simulink model "pmuReplay"  (R2018b)
settings: Solver=ode23tb  StartTime=0.0  StopTime=50  MaxStep=1/60  RelTol=1e-4  AbsTol=1e-3  EnableMultiTasking=on
PreLoadFcn:
  | addpath('PMU_Events');
  | load('PMU_ImportedData.mat')
InitFcn:
  | i = 3;
undefined symbols (not defined in the file): D1, Delta
libraries: powerlib x4, simulink x4, microgridLibrary x1, re_lib x1, powerlib_meascontrol x1
Description:
  | Copyright 2008-2017 The MathWorks, Inc.
settings Model: ExtModeAutoUpdateStatusClock=off  Creator=MathWorks  LastModifiedBy=jlesage
settings SolverCC: AutoScaleAbsTol=off
settings DataIOCC: LimitDataPoints=on  SaveFormat=StructureWithTime  SignalLoggingSaveFormat=ModelDataLogs  SaveOutput=off  SignalLogging=off  DSMLogging=off  SaveTime=off  SignalLoggingName=sigsOut
settings OptimizationCC: ExpressionDepthLimit=2147483647  InitFltsAndDblsToZero=on  EfficientMapNaN2IntZero=off  LifeSpan=inf
settings DebuggingCC: UnderspecifiedInitializationDetection=Classic  MergeDetectMultiDrivingBlocksExec=none  CheckExecutionContextPreStartOutputMsg=on  CheckExecutionContextRuntimeOutputMsg=on  SignalResolutionControl=TryResolveAllWithWarning  MultiTaskDSMMsg=warning  MultiTaskCondExecSysMsg=none  FcnCallInpInsideContextMsg=warning  UnconnectedLineMsg=none  StateNameClashWarn=warning  InitInArrayFormatMsg=none  SFUnexpectedBacktrackingDiag=warning  SFNoUnconditionalDefaultTransitionDiag=warning  SFExecutionAtInitializationDiag=none
settings HardwareCC: ProdBitPerPointer=32  ProdBitPerSizeT=32  ProdBitPerPtrDiffT=32  ProdLargestAtomicFloat=None  ProdIntDivRoundTo=Undefined  ProdEndianess=Unspecified  ProdWordSize=32  ProdHWDeviceType=32-bit Generic  TargetUnknown=on
settings ModelReferenceCC: PropagateSignalLabelsOutOfModel=off
settings SFSimCC: SimUseLocalCustomCode=off
settings RTWCC: RTWUseLocalCustomCode=off
settings CodeAppCC: StateflowObjectComments=on
settings GRTTargetCC: TargetLangStandard=C89/C90 (ANSI)  GeneratePreprocessorConditionals=Disable all  CombineOutputUpdateFcns=off  GRTInterface=on
settings ConfigComp: CovMetricSettings=dw  CovHtmlReporting=on  CovSaveCumulativeToWorkspaceVar=on  CovSaveSingleToWorkspaceVar=on  CovExternalEMLEnable=off  CovSFcnEnable=off
settings SimscapeCC: SimscapeNormalizeSystem=off

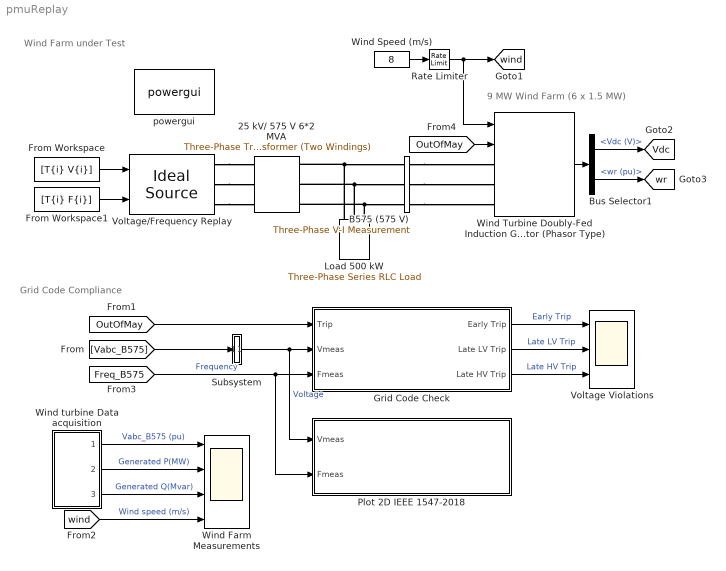
== system pmuReplay ==
  note: Wind Farm under Test
  note: Grid Code Compliance
  note: 9 MW Wind Farm
      | (6 x 1.5 MW)
  25 kV/ 575 V 6*2 MVA : powerlib/Elements/Three-Phase Transformer (Two Windings)  Winding1Connection=Yg  Winding2Connection=Delta (D1)  CoreType=Three single-phase transformers  SetSaturation=off  Hysteresis=off  DataFile='hysteresis'  SetInitialFlux=off  Measurements=None  UNITS=pu  NominalPower="[2e6*6  60]"  Winding1=[25e3 , 0.025/30 , 0.025]  Winding2=[ 575, 0.025/30 , 0.025]  Rm=500  Lm=inf  L0=0.5  Saturation=[ 0,0 ; 0.0024,1.2 ; 1.0,1.52 ]  InitialFluxes=[ 0.8 , -0.8 , 0.7 ]  MoreParameters=off  BreakLoop=off  DataType=off  TransfoNumber=0
      settings: SourceProductName=Simscape Electrical
  B575 (575 V) : powerlib/Measurements/Three-Phase V-I Measurement  VoltageMeasurement=phase-to-ground  SetLabelV=on  LabelV=Vabc_B575  Vpu=on  VpuLL=off  CurrentMeasurement=yes  SetLabelI=on  LabelI=Iabc_B575  Ipu=on  Pbase=6*1.5e6/0.9  Vbase=575  OutputType=Complex  PhasorSimulation=on  PSBequivalent=0
      settings: SourceProductName=Simscape Electrical
  Bus Selector1 : BusSelector  OutputSignals=Vdc (V),wr (pu)
  From Workspace : FromWorkspace  VariableName=[T{i} V{i}]  SampleTime=0  OutputAfterFinalValue=Holding final value
  From Workspace1 : FromWorkspace  VariableName=[T{i} F{i}]  SampleTime=0  OutputAfterFinalValue=Holding final value
  Grid Code Check : Subsystem  mask(Grid Code Compliance){curveSelect=IEEE 1547-2018, limitSelect=Only Mandatory, innerTimeLVRT=[-1, 0-1e-6, 0, 0.15-1e-6, 0.15, 0.3-1e-6, 0.3, 2-1e-6, 2, 3-1e-6, 3], innerMagLVRT=[0.9, 0.9, 0, 0, 0.45, 0.45, 0.65, 0.65, 0.75, 0.75, 0.9], innerTimeHVRT=[-1, 0-1e-6, 0, 0.2-1e-6, 0.2, 0.5-1e-6, 0.5, 1-1e-6, 1], innerMagHVRT=[1.1, 1.1, 1.2, 1.2, 1.175, 1.175, 1.15, 1.15, 1.1], outerTimeLVRT=[-1, 0-1e-6, 0, 0.15-1e-6, 0.15, 0.3-1e-6, 0.3, 2-1e-6, 2, 3-1e-6, 3], outerMagLVRT=[0.9, 0.9, 0, 0, 0.45, 0.45, 0.65, 0.65, 0.75, 0.75, 0.9], outerTimeHVRT=[-1, 0-1e-6, 0, 0.2-1e-6, 0.2, 0.5-1e-6, 0.5, 1-1e-6, 1], outerMagHVRT=[1.1, 1.1, 1.2, 1.2, 1.175, 1.175, 1.15, 1.15, 1.1], resetTime=50, buffer=0.02}
      mask prompts: curveSelect "Voltage Grid Code"; limitSelect "Custom Grid Code Limits"; innerTimeLVRT "Low Limit Time (s)"; innerMagLVRT "Low Limit Magnitude (pu)"; innerTimeHVRT "High Limit Time (s)"; innerMagHVRT "High Limit Magnitude (pu)"; outerTimeLVRT "Low Limit Time (s)"; outerMagLVRT "Low Limit Magnitude (pu)"; outerTimeHVRT "High Limit Time (s)"; outerMagHVRT "High Limit Magnitude (pu)"; resetTime "Reset Time for Events (s)"; buffer "Trip Buffer Time (s)"
      mask help: This block detects grid events and plots the selected grid code.
      mask init:
      | % PRC-024 Definition
      | PRC024_LV_T = [-1, 0-1e-6, 0, 0.15-1e-6, 0.15, 0.3-1e-6, 0.3, 2-1e-6, 2, 3-1e-6, 3];
      | PRC024_LV_V = [0.9, 0.9, 0, 0, 0.45, 0.45, 0.65, 0.65, 0.75, 0.75, 0.9];
      | PRC024_HV_T = [-1, 0-1e-6, 0, 0.2-1e-6, 0.2, 0.5-1e-6, 0.5, 1-1e-6, 1];
      | PRC024_HV_V = [1.1, 1.1, 1.2, 1.2, 1.175, 1.175, 1.15, 1.15, 1.1];
      | 
      | % ERCOT Definition
      | ERCOT_LV_T = [-1 0-1e-6 0 0.15 1.75 2 600-1e-6 600];
      | ERCOT_LV_V = [0.95 0.95 0 0 0.9 0.9 0.9 0.95];
      | ERCOT_HV_T = [-1 0-1e-6	0 0.2-1e-6 0.2 0.5-1e-6	0.5	1-1e-6 1 600-1e-6 600];
      | ERCOT_HV_V = [1.1 1.1 1.2 1.2 1.175 1.175 1.15 1.15	1.1	1.1	1.1];
      | 
      | % IEEE 1547-2018
      | IEEE1547_LV_T_out = [-1 0-1e-6 0 0.16-1e-6 0.16 10-1e-6 10 1000-1e-6 1000];
      | IEEE1547_LV_V_out = [0.88 0.88 0 0 0.45 0.45 0.7 0.7 0.88];
      | IEEE1547_HV_T_out = [-1 0-1e-6 0 0.16-1e-6 0.16 10-1e-6 10 1000];
      | IEEE1547_HV_V_out = [1.1 1.1 1.3 1.3 1.2 1.2 1.15 1.1];
      | 
      | IEEE1547_LV_T_in = [-1 0-1e-6 0 0.16-1e-6 0.16 0.32-1e-6 0.32 3 5 1000];
      | IEEE1547_LV_V_in = [0.88 0.88 0.3 0.3 0.45 0.45 0.65 0.65 0.88 0.88];
      | IEEE1547_HV_T_in = [-1 0-1e-6 0 0.2-1e-6 0.2 0.5-1e-6 0.5 1-1e-6 1 600-1e-6 600];
      | IEEE1547_HV_V_in = [1.1 1.1 1.2 1.2 1.175 1.175 1.15 1.15 1.1 1.1 1.1];
      | 
      | % PRC-024: WECC Definition
      | WECC_LF_T = [-1, 0-1e-6, 0, 0.75-1e-6, 0.75, 7.5-1e-6, 7.5, 30-1e-6, 30, 180-1e-6, 180 10000];
      | WECC_LF_F = [59.4, 59.4, 57, 57, 57.3, 57.3, 57.8, 57.8, 58.4, 58.4, 59.4 59.4];
      | WECC_HF_T = [-1, 0-1e-6, 0, 30-1e-6, 30, 180-1e-6, 180, 10000];
      | WECC_HF_F = [60.6, 60.6, 61.7, 61.7, 61.6, 61.6, 60.6, 60.6];
      | 
      | % PRC-024: ERCOT Definition
      | ERCOT_LF_T = [-1, 0-1e-6, 0, 2-1e-6, 2, 30-1e-6, 30, 540-1e-6, 540, 10000];
      | ERCOT_LF_F = [59.4, 59.4, 57.5, 57.5, 58, 58, 58.4, 58.4, 59.4, 59.4];
      | ERCOT_HF_T = [-1, 0-1e-6, 0, 30-1e-6, 30, 540-1e-6, 540, 10000];
      | ERCOT_HF_F = [60.6, 60.6, 61.8, 61.8, 61.6, 61.6, 60.6, 60.6];
      | 
      | % PRC-024: East Definition
      | East_LF_T = [-1, 0-1e-6, 0, 2-1e-6, 1800, 10000];
      | East_LF_F = [59.5, 59.5, 57.8, 57.8, 59.5, 59.5];
      | East_HF_T = [-1, 0-1e-6, 0, 2-1e-6, 600, 10000];
      | East_HF_F = [60.5, 60.5, 62.2, 62.2, 60.5, 60.5];
      | 
      | % PRC-024: Quebec Definition
      | Quebec_LF_T = [-1, 0-1e-6, 0, 0.35-1e-6, 0.35, 2-1e-6, 2, 10-1e-6, 10, 90-1e-6, 90, 660-1e-6, 660 10000];
      | Quebec_LF_F = [59.4, 59.4, 55.5, 55.5, 56.5, 56.5, 57, 57, 57.5, 57.5, 58.5, 58.5, 59.4, 59.4];
      | Quebec_HF_T = [-1, 0-1e-6, 0, 5-1e-6, 5, 90-1e-6, 90, 660-1e-6, 660, 10000];
      | Quebec_HF_F = [60.6, 60.6, 66, 66, 63, 63, 61.5, 61.5, 60.6, 60.6];
      | 
      | % IEEE 1547-2018
      | IEEE1547_LF_T_out = [-1, 0-1e-6, 0, 0.16-1e-6, 0.16, 300-1e-6, 300, 10000];
      | IEEE1547_LF_F_out = [58.5, 58.5, 50, 50, 56.5, 56.5, 58.5, 58.5];
      | IEEE1547_HF_T_out = [-1, 0-1e-6, 0, 0.16-1e-6, 0.16, 300-1e-6, 300, 1000-1e-6, 1000, 10000];
      | IEEE1547_HF_F_out = [60.6, 60.6, 66, 66, 62, 62, 61, 61, 60.6, 60.6];
      | 
      | IEEE1547_LF_T_in = [-1, 0-1e-6, 0, 299-1e-6, 299, 10000];
      | IEEE1547_LF_F_in = [58.5, 58.5, 57, 57, 58.5, 58.5];
      | IEEE1547_HF_T_in = [-1, 0-1e-6, 0, 299-1e-6, 299, 10000];
      | IEEE1547_HF_F_in = [60.6, 60.6, 62, 62, 60.6, 60.6];
      | 
      | 
      | % Disable Options depending on selection
      | currentEnables = get_param(gcb,'MaskEnables');
      | if strcmp(curveSelect,'Custom Limit')
      |     for i = 2:10
      |         if i <= 6
      |             currentEnables{i} = 'on';
      |         elseif i > 6 && strcmp(limitSelect,'Mandatory/Optional Limits')
      |             currentEnables{i} = 'on';
      |         else
      |             currentEnables{i} = 'off';
      |         end
      |     end
      | else
      |     for i = 2:10
      |         currentEnables{i} = 'off';
      |     end
      | end
      | set_param(gcb,'MaskEnables',currentEnables);
      | 
      | % Setup Vectors
      | if strcmp(curveSelect,'Custom Limit')
      |     inLV_T = innerTimeLVRT; inHV_T = innerTimeHVRT;   
      |     inLV_V = innerMagLVRT;  inHV_V = innerMagHVRT;
      |     outLV_T = outerTimeLVRT;outHV_T = outerTimeHVRT;
      |     outLV_V = outerMagLVRT; outHV_V = outerMagHVRT;
      |     
      |     inLF_T = innerTimeLFRT; inHF_T = innerTimeHFRT;   
      |     inLF_F = innerMagLFRT;  inHF_F = innerMagHFRT;
      |     outLF_T = outerTimeLFRT;outHF_T = outerTimeHFRT;
      |     outLF_F = outerMagLFRT; outHF_F = outerMagHFRT;
      | elseif strcmp(curveSelect,'ERCOT')
      |     inLV_T = ERCOT_LV_T;   inHV_T = ERCOT_HV_T;   
      |     inLV_V = ERCOT_LV_V;   inHV_V = ERCOT_HV_V;
      |     outLV_T = ERCOT_LV_T;  outHV_T = ERCOT_HV_T;
      |     outLV_V = ERCOT_LV_V;  outHV_V = ERCOT_HV_V;
      |     
      |     inLF_T = ERCOT_LF_T;   inHF_T = ERCOT_HF_T;   
      |     inLF_F = ERCOT_LF_F;   inHF_F = ERCOT_HF_F;
      |     outLF_T = ERCOT_LF_T;  outHF_T = ERCOT_HF_T;
      |     outLF_F = ERCOT_LF_F;  outHF_F = ERCOT_HF_F;
      | elseif strcmp(curveSelect,'IEEE 1547-2018')
      |     inLV_T = IEEE1547_LV_T_in;   inHV_T = IEEE1547_HV_T_in;   
      |     inLV_V = IEEE1547_LV_V_in;   inHV_V = IEEE1547_HV_V_in;
      |     outLV_T = IEEE1547_LV_T_out;  outHV_T = IEEE1547_HV_T_out;
      |     outLV_V = IEEE1547_LV_V_out;  outHV_V = IEEE1547_HV_V_out;
      |     
      |     inLF_T = IEEE1547_LF_T_in;   inHF_T = IEEE1547_HF_T_in;   
      |     inLF_F = IEEE1547_LF_F_in;   inHF_F = IEEE1547_HF_F_in;
      |     outLF_T = IEEE1547_LF_T_out;  outHF_T = IEEE1547_HF_T_out;
      |     outLF_F = IEEE1547_LF_F_out;  outHF_F = IEEE1547_HF_F_out;
      | else    
      |     inLV_T = PRC024_LV_T;   inHV_T = PRC024_HV_T;   
      |     inLV_V = PRC024_LV_V;   inHV_V = PRC024_HV_V;
      |     outLV_T = PRC024_LV_T;  outHV_T = PRC024_HV_T;
      |     outLV_V = PRC024_LV_V;  outHV_V = PRC024_HV_V;
      | end
      | 
      | if buffer > 0
      |     inLV_T = inLV_T - [zeros(1,3) buffer/2*ones(1,numel(inLV_T)-3)];
      |     inHV_T = inHV_T - [zeros(1,3) buffer/2*ones(1,numel(inHV_T)-3)];
      |     outLV_T = outLV_T + [zeros(1,3) buffer/2*ones(1,numel(outLV_T)-3)];
      |     outHV_T = outHV_T + [zeros(1,3) buffer/2*ones(1,numel(outHV_T)-3)];
      | end
      mask TypeOptions curveSelect: ERCOT | IEEE 1547-2018 | Custom Limit
      mask TypeOptions limitSelect: Only Mandatory | Mandatory/Optional Limits
      mask DialogControl Container6 Prompt: Custom Grid Code Specification
      mask DialogControl Container5 Prompt: Mandatory (Inner) Limit
      mask DialogControl Container7 Prompt: Optional (Outer) Limit
      mask Display:
      | color('blue');disp(['Grid Code Check\n' curveSelect])
      | color('black');
      | port_label('input',1,'Trip')
      | port_label('input',2,'V (pu)')
      | port_label('input',3,'Freq (Hz)')
      | 
      | port_label('output',1,'Early Trip')
      | port_label('output',2,'Late LV Trip')
      | port_label('output',3,'Late HV Trip')
  Load 500 kW : powerlib/Elements/Three-Phase Series RLC Load  LConnTagsString=A|B|C  Configuration=Y (grounded)  NominalVoltage=575  Vabc=[1e3 1e3 1e3]  Vabcp=[1e3 1e3 1e3]  NominalFrequency=60  UnbalancedPower=off  ActivePower=500e3  InductivePower=0  CapacitivePower=0  Pabc=[10e3 9e3 11e3]  QLabc=[100 90 110]  QCabc=[100 90 110]  Pabcp=[10e3 9e3 11e3]  QLabcp=[100 90 110]  QCabcp=[100 90 110]  Measurements=None  LoadType=constant Z
      settings: SourceProductName=Simscape Electrical
  Plot 2D IEEE 1547-2018 : Subsystem
      mask Display:
      | color('blue');disp('IEEE 1547-2018\n Voltage vs. Frequency')
      | color('black');
      | port_label('input',1,'V (pu)')
      | port_label('input',2,'Freq (Hz)')
  Rate Limiter : RateLimiter
  Subsystem : Subsystem
  Voltage Violations : Scope  NumInputPorts=3
  Voltage/Frequency Replay : microgridLibrary/Ideal Source  InternalConnection=Yg  VoltagePhases=off  Voltage=25e3  PhaseAngle=0  Voltage_phases=[25e3 25e3 25e3]/sqrt(3)  PhaseAngles_phases=[0 -120 +120]  Frequency=60  NonIdealSource=off  SpecifyImpedance=off  Resistance=0.8929  Inductance=16.58e-3  ShortCircuitLevel=100e6  BaseVoltage=25e3  XRratio=7  BusType=swing  Pref=10e3  Qref=0  Prefabc=[10e3, 10e3, 10e3]  Qrefabc=[0, 0, 0]  Qmin=-inf  Qmax=inf
  Wind Speed (m/s) : Constant  Value=8
  Wind Farm Measurements : Scope  NumInputPorts=4
  Wind Turbine Doubly-Fed Induction Generator (Phasor Type) : re_lib/Wind Generation/Wind Turbine Doubly-Fed Induction Generator (Phasor Type)  ExternalTm=off  nom=[6*1.5e6 575 60]  sta=[ 0.00706 0.171]  rot=[ 0.005 0.156]  Lm=2.9  mec=[5.04 0.01 3]  init=[0.2 0 0 0 0 0]  speed_power=[0 0; 0.24 0.007; 0.36 0.024; 0.6 0.112; 0.96 0.46; 1.2 0.898; 1.5 0.898]  Pmec=6*1.5e6  speed_ABCD=[0.7 0.71 1.2 1.21]  power_C=0.73  wind_point_C=12  pitch_gain=500  pitch_max=45  pitch_rate=2  Pmax=0.5  Lchoke=[0.15 0.15/100]  init_inductor=[0 90]  Vdc_nom=1200  capacitor=6*10000e-6  ControlVQ=Voltage regulation  Vref=1.0  ExternalVref=off  Qref=0  ExternalQref=off  Iq_ref=0  ExternalIqref=off  Kpi_volt_reg=[1.25 300]  Xs=0.02  Kpi_Q=[0.05 5]  Kpi_power_reg=[1 100]  Kpi_dc_reg=[0.002 0.05]  Kpi_grid_side_cur_reg=[1 100]  Kpi_rotor_side_cur_reg=[0.3 8]  V_slew_rate=100  Q_slew_rate=100  power_slew_rate=1  current_slew_rate=200
      settings: SourceProductName=Simscape Electrical  SourceProductBaseCode=PS
  Wind turbine Data acquisition : Subsystem
  powergui : powerlib/powergui  Priority=2  SimulationMode=Phasor  SampleTime=0  frequency=60  Iterations=50  frequencyindice=60  Pbase=100e6  ErrMax=1e-4  UnitsV=kV  UnitsW=MW  buscounter=0  FunctionMessages=off  echomessages=off  EnableUseOfTLC=off  CurrentSourceSwitches=off  DisableSnubberDevices=off  DisableRonSwitches=off  DisableVfSwitches=off  DisplayEquations=off  SolverType=Tustin  Interpol=off  ExternalGateDelay=off  methode=off  Ts=0  x0status=blocks  SPID=off  SwTol=0  HookPort=off  RestoreLinks=warning  ResistiveCurrentMeasurement=off  Frange=[0:2:500]  Ylog=off  Xlog=off  ShowGrid=off  save=off  variable=ZData  structure=0  ZoomFFT=on  StartTime=0.0  cycles=1  DisplayStyle=1  fundamental=60  FreqAxis=off  MaxFrequency=1000  frequencyindicesteady=1  RmsSteady=1  display=off
  tag scope: Vdc=global, wind=global, wr=global
  wires:
  Bus Selector1/1 -> [Vdc]  "<Vdc (V)>"
  Bus Selector1/2 -> [wr]  "<wr (pu)>"
  Wind Turbine Doubly-Fed Induction Generator (Phasor Type)/1 -> Bus Selector1/1
  Wind Speed (m/s)/1 -> Rate Limiter/1
  Rate Limiter/1 -> Wind Turbine Doubly-Fed Induction Generator (Phasor Type)/1, [wind]
  [OutOfMay] -> Grid Code Check/1(Trip)
  Grid Code Check/1(Early Trip) -> Voltage Violations/1  "Early Trip"
  Grid Code Check/2(Late LV Trip) -> Voltage Violations/2  "Late LV Trip"
  Grid Code Check/3(Late HV Trip) -> Voltage Violations/3  "Late HV Trip"
  [Vabc_B575] -> Subsystem/1(V (pu))
  From Workspace/1 -> Voltage/Frequency Replay/1
  From Workspace1/1 -> Voltage/Frequency Replay/2
  Subsystem/1(V) -> Plot 2D IEEE 1547-2018/1(Vmeas), Grid Code Check/2(Vmeas)  "Voltage"
  [wind] -> Wind Farm Measurements/4  "Wind speed (m/s)"
  Wind turbine Data acquisition/3(Q_mean) -> Wind Farm Measurements/3  "Generated Q(Mvar)"
  Wind turbine Data acquisition/2(P_mean) -> Wind Farm Measurements/2  "Generated P(MW)"
  Wind turbine Data acquisition/1(V_turbine) -> Wind Farm Measurements/1  "Vabc_B575 (pu)"
  [Freq_B575] -> Plot 2D IEEE 1547-2018/2(Fmeas), Grid Code Check/3(Fmeas)  "Frequency"
  [OutOfMay] -> Wind Turbine Doubly-Fed Induction Generator (Phasor Type)/2
  connections:
  Load 500 kW/LConn2 -- B575 (575 V)/LConn2 -- 25 kV/ 575 V 6*2 MVA/RConn2
  Load 500 kW/LConn1 -- B575 (575 V)/LConn1 -- 25 kV/ 575 V 6*2 MVA/RConn1
  Load 500 kW/LConn3 -- B575 (575 V)/LConn3 -- 25 kV/ 575 V 6*2 MVA/RConn3
  B575 (575 V)/RConn1 -- Wind Turbine Doubly-Fed Induction Generator (Phasor Type)/LConn1
  B575 (575 V)/RConn2 -- Wind Turbine Doubly-Fed Induction Generator (Phasor Type)/LConn2
  B575 (575 V)/RConn3 -- Wind Turbine Doubly-Fed Induction Generator (Phasor Type)/LConn3
  Voltage/Frequency Replay/RConn1 -- 25 kV/ 575 V 6*2 MVA/LConn1
  Voltage/Frequency Replay/RConn2 -- 25 kV/ 575 V 6*2 MVA/LConn2
  Voltage/Frequency Replay/RConn3 -- 25 kV/ 575 V 6*2 MVA/LConn3

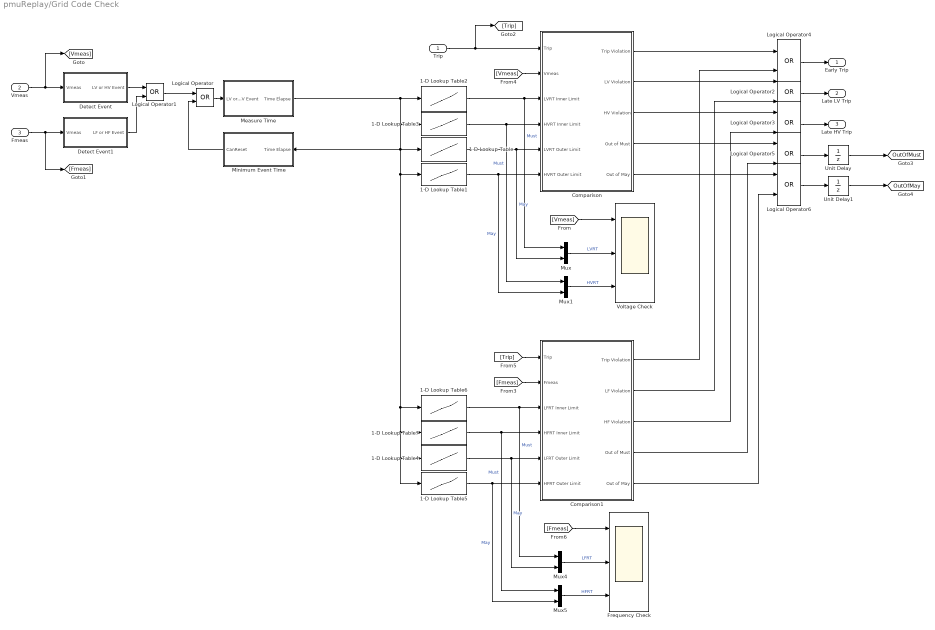
== system pmuReplay/Grid Code Check ==
  Trip : Inport
  Vmeas : Inport  Port=2
  Fmeas : Inport  Port=3
  1-D Lookup Table : Lookup_n-D  NumberOfTableDimensions=1  BreakpointsForDimension1=outLV_T  Table=outLV_V  ExtrapMethod=Clip  InternalRulePriority=Speed  RndMeth=Simplest  InputSameDT=on
  1-D Lookup Table1 : Lookup_n-D  NumberOfTableDimensions=1  BreakpointsForDimension1=outHV_T  Table=outHV_V  ExtrapMethod=Clip  InternalRulePriority=Speed  RndMeth=Simplest  InputSameDT=on
  1-D Lookup Table2 : Lookup_n-D  NumberOfTableDimensions=1  BreakpointsForDimension1=inLV_T  Table=inLV_V  ExtrapMethod=Clip  InternalRulePriority=Speed  RndMeth=Simplest  InputSameDT=on
  1-D Lookup Table3 : Lookup_n-D  NumberOfTableDimensions=1  BreakpointsForDimension1=inHV_T  Table=inHV_V  ExtrapMethod=Clip  InternalRulePriority=Speed  RndMeth=Simplest  InputSameDT=on
  1-D Lookup Table4 : Lookup_n-D  NumberOfTableDimensions=1  BreakpointsForDimension1=outLF_T  Table=outLF_F  ExtrapMethod=Clip  InternalRulePriority=Speed  RndMeth=Simplest  InputSameDT=on
  1-D Lookup Table5 : Lookup_n-D  NumberOfTableDimensions=1  BreakpointsForDimension1=outHF_T  Table=outHF_F  ExtrapMethod=Clip  InternalRulePriority=Speed  RndMeth=Simplest  InputSameDT=on
  1-D Lookup Table6 : Lookup_n-D  NumberOfTableDimensions=1  BreakpointsForDimension1=inLF_T  Table=inLF_F  ExtrapMethod=Clip  InternalRulePriority=Speed  RndMeth=Simplest  InputSameDT=on
  1-D Lookup Table7 : Lookup_n-D  NumberOfTableDimensions=1  BreakpointsForDimension1=inHF_T  Table=inHF_F  ExtrapMethod=Clip  InternalRulePriority=Speed  RndMeth=Simplest  InputSameDT=on
  Comparison : Subsystem
  Comparison1 : Subsystem
  Detect Event : Subsystem
  Detect Event1 : Subsystem
  Frequency Check : Scope  NumInputPorts=3
  Logical Operator{,1..6} (7 alike) : Logic  Operator=OR  AllPortsSameDT=off  OutDataTypeStr=boolean
  Measure Time : Subsystem
  Minimum Event Time : Subsystem
  Mux{,1,4..5} (4 alike) : Mux  Inputs=2
  Unit Delay : UnitDelay  SampleTime=-1
  Unit Delay1 : UnitDelay  SampleTime=-1
  Voltage Check : Scope  NumInputPorts=3
  Early Trip : Outport
  Late LV Trip : Outport  Port=2
  Late HV Trip : Outport  Port=3
  tag scope: OutOfMay=global, OutOfMust=global
  wires:
  Trip/1 -> [Trip], Comparison/1(Trip)
  [Vmeas] -> Comparison/2(Vmeas)
  1-D Lookup Table1/1 -> Mux1/2, Comparison/6(HVRT Outer Limit)  "May"
  1-D Lookup Table/1 -> Mux/2, Comparison/5(LVRT Outer Limit)  "May"
  Vmeas/1 -> [Vmeas], Detect Event/1(Vmeas)
  1-D Lookup Table2/1 -> Mux/1, Comparison/3(LVRT Inner Limit)  "Must"
  1-D Lookup Table3/1 -> Mux1/1, Comparison/4(HVRT Inner Limit)  "Must"
  Mux/1 -> Voltage Check/2  "LVRT"
  Mux1/1 -> Voltage Check/3  "HVRT"
  [Vmeas] -> Voltage Check/1
  Logical Operator/1 -> Measure Time/1(LV or HV Event)
  Minimum Event Time/1(CanReset) -> Logical Operator/2
  [Fmeas] -> Comparison1/2(Fmeas)
  Fmeas/1 -> Detect Event1/1(Vmeas), [Fmeas]
  Measure Time/1(Time Elapse) -> 1-D Lookup Table6/1, 1-D Lookup Table7/1, 1-D Lookup Table4/1, 1-D Lookup Table5/1, 1-D Lookup Table1/1, Minimum Event Time/1(Time Elapse), 1-D Lookup Table/1, 1-D Lookup Table3/1, 1-D Lookup Table2/1
  [Trip] -> Comparison1/1(Trip)
  Comparison/1(Trip Violation) -> Logical Operator4/1
  Logical Operator4/1 -> Early Trip/1
  Comparison1/1(Trip Violation) -> Logical Operator4/2
  Logical Operator2/1 -> Late LV Trip/1
  Logical Operator3/1 -> Late HV Trip/1
  Comparison/2(LV Violation) -> Logical Operator2/1
  Comparison/3(HV Violation) -> Logical Operator3/1
  Comparison1/3(HF Violation) -> Logical Operator3/2
  Comparison1/2(LF Violation) -> Logical Operator2/2
  [Fmeas] -> Frequency Check/1
  Mux5/1 -> Frequency Check/3  "HFRT"
  Mux4/1 -> Frequency Check/2  "LFRT"
  1-D Lookup Table7/1 -> Mux5/1, Comparison1/4(HFRT Inner Limit)  "Must"
  1-D Lookup Table6/1 -> Mux4/1, Comparison1/3(LFRT Inner Limit)  "Must"
  1-D Lookup Table4/1 -> Mux4/2, Comparison1/5(LFRT Outer Limit)  "May"
  1-D Lookup Table5/1 -> Mux5/2, Comparison1/6(HFRT Outer Limit)  "May"
  Detect Event/1(LV or HV Event) -> Logical Operator1/1
  Detect Event1/1(LF or HF Event) -> Logical Operator1/2
  Logical Operator1/1 -> Logical Operator/1
  Comparison/4(Out of Must) -> Logical Operator5/1
  Comparison1/4(Out of Must) -> Logical Operator5/2
  Logical Operator5/1 -> Unit Delay/1
  Unit Delay/1 -> [OutOfMust]
  Comparison/5(Out of May) -> Logical Operator6/1
  Logical Operator6/1 -> Unit Delay1/1
  Comparison1/5(Out of May) -> Logical Operator6/2
  Unit Delay1/1 -> [OutOfMay]

== system pmuReplay/Plot 2D IEEE 1547-2018 ==
  Vmeas : Inport
  Fmeas : Inport  Port=2
  Clock : Clock
  MATLAB Function : MATLAB Function  TreatAsAtomicUnit=on  SystemSampleTime=0.1
  wires:
  Fmeas/1 -> MATLAB Function/2(F)
  Clock/1 -> MATLAB Function/3(t)
  Vmeas/1 -> MATLAB Function/1(V)

== system pmuReplay/Subsystem ==
  V (pu) : Inport
  Clock : Clock
  Compare To Constant : simulink/Logic and Bit Operations/Compare To Constant  relop=>=  const=5  OutDataTypeStr=boolean
  "Complex to Magnitude-Angle " : ComplexToMagnitudeAngle  Output=Magnitude
  Constant2 : Constant
  Selector : Selector  InputPortWidth=3  IndexOptions=Index vector (dialog)  Indices=[1]  OutputSizes=1
  Switch : Switch  Criteria=u2 > Threshold
  V : Outport
  wires:
  Clock/1 -> Compare To Constant/1
  Compare To Constant/1 -> Switch/2
  Switch/1 -> V/1
  Constant2/1 -> Switch/3
  "Complex to Magnitude-Angle "/1 -> Selector/1
  V (pu)/1 -> "Complex to Magnitude-Angle "/1
  Selector/1 -> Switch/1

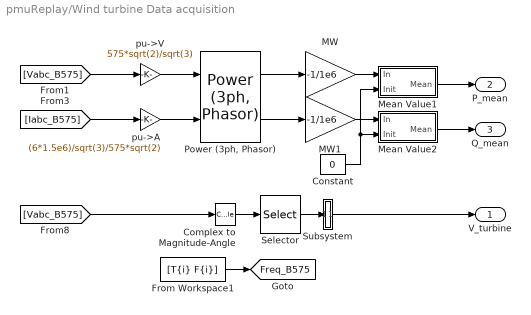
== system pmuReplay/Wind turbine Data acquisition ==
  "Complex to Magnitude-Angle " : ComplexToMagnitudeAngle  Output=Magnitude
  Constant : Constant  Value=0
  From Workspace1 : FromWorkspace  VariableName=[T{i} F{i}]  SampleTime=0  OutputAfterFinalValue=Holding final value
  MW : Gain  Gain=-1/1e6  SaturateOnIntegerOverflow=on  OutDataTypeStr=Inherit: Same as input  ParamDataTypeStr=Inherit: Same as input
  MW1 : Gain  Gain=-1/1e6  SaturateOnIntegerOverflow=on  OutDataTypeStr=Inherit: Same as input  ParamDataTypeStr=Inherit: Same as input
  Mean Value1 : Subsystem  mask(Mean value){Period=1/60}
      mask prompts: Period "Averaging period (s):"
      mask help: This block uses the running window averaging technique to compute the mean value of the input signal over the specified period.
  Mean Value2 : Subsystem  mask(Mean value){Period=1/60}
      mask prompts: Period "Averaging period (s):"
      mask help: This block uses the running window averaging technique to compute the mean value of the input signal over the specified period.
  "Power (3ph, Phasor)" : powerlib_meascontrol/Measurements/Power (3ph, Phasor)
      settings: SourceProductName=Simscape Electrical  SourceProductBaseCode=PS
  Selector : Selector  InputPortWidth=3  IndexOptions=Index vector (dialog)  Indices=[1]  OutputSizes=1
  Subsystem : Subsystem
  pu->A : Gain  Gain=(6*1.5e6)/sqrt(3)/575*sqrt(2)  SaturateOnIntegerOverflow=on  OutDataTypeStr=Inherit: Same as input  ParamDataTypeStr=Inherit: Same as input
  pu->V : Gain  Gain=575*sqrt(2)/sqrt(3)  SaturateOnIntegerOverflow=on  OutDataTypeStr=Inherit: Same as input  ParamDataTypeStr=Inherit: Same as input
  V_turbine : Outport
  P_mean : Outport  Port=2
  Q_mean : Outport  Port=3
  tag scope: Freq_B575=global
  wires:
  [Iabc_B575] -> pu->A/1
  [Vabc_B575] -> pu->V/1
  pu->A/1 -> "Power (3ph, Phasor)"/2
  pu->V/1 -> "Power (3ph, Phasor)"/1
  MW/1 -> Mean Value1/1(In)
  MW1/1 -> Mean Value2/1(In)
  Mean Value1/1(Mean) -> P_mean/1
  Mean Value2/1(Mean) -> Q_mean/1
  Constant/1 -> Mean Value1/2(Init), Mean Value2/2(Init)
  "Power (3ph, Phasor)"/1 -> MW/1
  "Power (3ph, Phasor)"/2 -> MW1/1
  "Complex to Magnitude-Angle "/1 -> Selector/1
  Selector/1 -> Subsystem/1(V (pu))
  Subsystem/1(V) -> V_turbine/1
  [Vabc_B575] -> "Complex to Magnitude-Angle "/1
  From Workspace1/1 -> [Freq_B575]

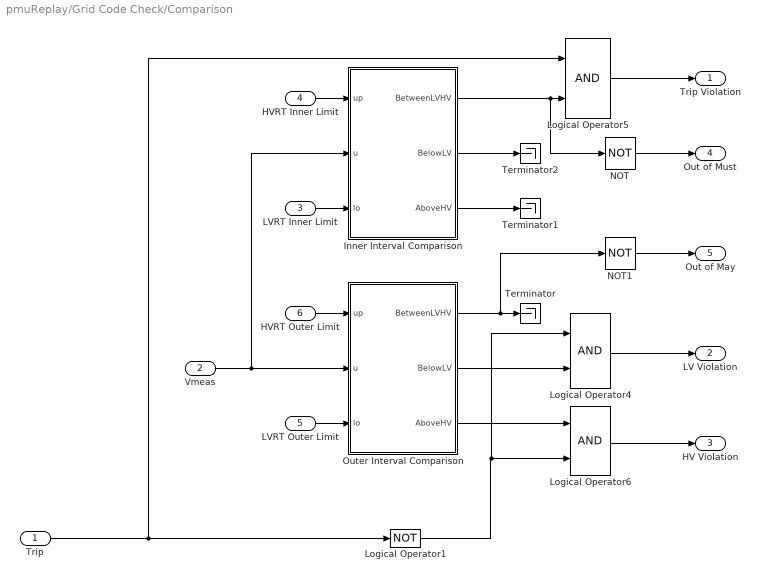
== system pmuReplay/Grid Code Check/Comparison ==
  Trip : Inport
  Vmeas : Inport  Port=2
  LVRT Inner Limit : Inport  Port=3
  HVRT Inner Limit : Inport  Port=4
  LVRT Outer Limit : Inport  Port=5
  HVRT Outer Limit : Inport  Port=6
  Inner Interval Comparison : Subsystem
  Logical Operator1 : Logic  Operator=NOT  AllPortsSameDT=off  OutDataTypeStr=boolean
  Logical Operator4 : Logic  AllPortsSameDT=off  OutDataTypeStr=boolean
  Logical Operator5 : Logic  AllPortsSameDT=off  OutDataTypeStr=boolean
  Logical Operator6 : Logic  AllPortsSameDT=off  OutDataTypeStr=boolean
  NOT : Logic  Operator=NOT  AllPortsSameDT=off  OutDataTypeStr=boolean
  NOT1 : Logic  Operator=NOT  AllPortsSameDT=off  OutDataTypeStr=boolean
  Outer Interval Comparison : Subsystem
  Terminator : Terminator
  Terminator1 : Terminator
  Terminator2 : Terminator
  Trip Violation : Outport
  LV Violation : Outport  Port=2
  HV Violation : Outport  Port=3
  Out of Must : Outport  Port=4
  Out of May : Outport  Port=5
  wires:
  Logical Operator5/1 -> Trip Violation/1
  Vmeas/1 -> Inner Interval Comparison/2(u), Outer Interval Comparison/2(u)
  LVRT Outer Limit/1 -> Outer Interval Comparison/3(lo)
  HVRT Outer Limit/1 -> Outer Interval Comparison/1(up)
  Outer Interval Comparison/2(BelowLV) -> Logical Operator4/2
  Outer Interval Comparison/3(AboveHV) -> Logical Operator6/1
  Logical Operator4/1 -> LV Violation/1
  Logical Operator6/1 -> HV Violation/1
  LVRT Inner Limit/1 -> Inner Interval Comparison/3(lo)
  HVRT Inner Limit/1 -> Inner Interval Comparison/1(up)
  Inner Interval Comparison/1(BetweenLVHV) -> NOT/1, Logical Operator5/2
  Outer Interval Comparison/1(BetweenLVHV) -> NOT1/1, Terminator/1
  Inner Interval Comparison/3(AboveHV) -> Terminator1/1
  Inner Interval Comparison/2(BelowLV) -> Terminator2/1
  Trip/1 -> Logical Operator5/1, Logical Operator1/1
  Logical Operator1/1 -> Logical Operator4/1, Logical Operator6/2
  NOT/1 -> Out of Must/1
  NOT1/1 -> Out of May/1

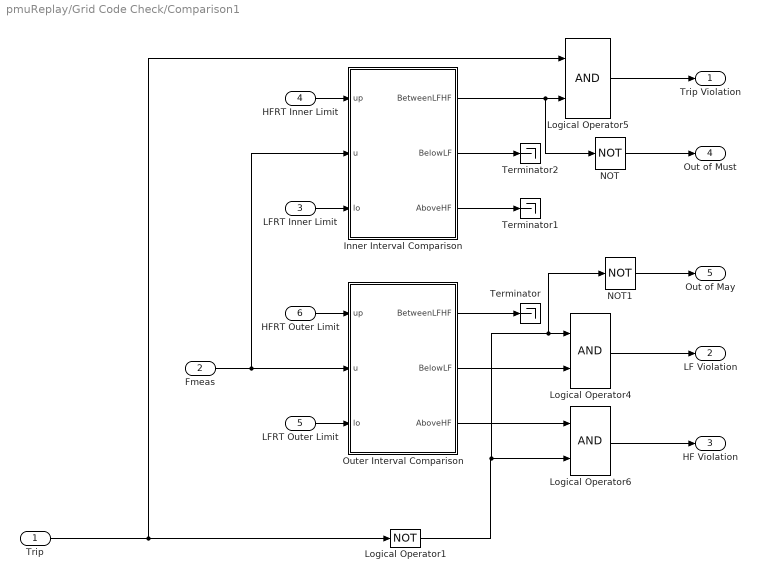
== system pmuReplay/Grid Code Check/Comparison1 ==
  Trip : Inport
  Fmeas : Inport  Port=2
  LFRT Inner Limit : Inport  Port=3
  HFRT Inner Limit : Inport  Port=4
  LFRT Outer Limit : Inport  Port=5
  HFRT Outer Limit : Inport  Port=6
  Inner Interval Comparison : Subsystem
  Logical Operator1 : Logic  Operator=NOT  AllPortsSameDT=off  OutDataTypeStr=boolean
  Logical Operator4 : Logic  AllPortsSameDT=off  OutDataTypeStr=boolean
  Logical Operator5 : Logic  AllPortsSameDT=off  OutDataTypeStr=boolean
  Logical Operator6 : Logic  AllPortsSameDT=off  OutDataTypeStr=boolean
  NOT : Logic  Operator=NOT  AllPortsSameDT=off  OutDataTypeStr=boolean
  NOT1 : Logic  Operator=NOT  AllPortsSameDT=off  OutDataTypeStr=boolean
  Outer Interval Comparison : Subsystem
  Terminator : Terminator
  Terminator1 : Terminator
  Terminator2 : Terminator
  Trip Violation : Outport
  LF Violation : Outport  Port=2
  HF Violation : Outport  Port=3
  Out of Must : Outport  Port=4
  Out of May : Outport  Port=5
  wires:
  Trip/1 -> Logical Operator1/1, Logical Operator5/1
  Inner Interval Comparison/2(BelowLF) -> Terminator2/1
  Inner Interval Comparison/3(AboveHF) -> Terminator1/1
  Outer Interval Comparison/1(BetweenLFHF) -> Terminator/1
  Inner Interval Comparison/1(BetweenLFHF) -> Logical Operator5/2, NOT/1
  HFRT Inner Limit/1 -> Inner Interval Comparison/1(up)
  LFRT Inner Limit/1 -> Inner Interval Comparison/3(lo)
  Logical Operator6/1 -> HF Violation/1
  Logical Operator4/1 -> LF Violation/1
  Outer Interval Comparison/3(AboveHF) -> Logical Operator6/1
  Outer Interval Comparison/2(BelowLF) -> Logical Operator4/2
  HFRT Outer Limit/1 -> Outer Interval Comparison/1(up)
  LFRT Outer Limit/1 -> Outer Interval Comparison/3(lo)
  Fmeas/1 -> Outer Interval Comparison/2(u), Inner Interval Comparison/2(u)
  Logical Operator5/1 -> Trip Violation/1
  NOT/1 -> Out of Must/1
  Logical Operator1/1 -> Logical Operator6/2, Logical Operator4/1, NOT1/1
  NOT1/1 -> Out of May/1

== system pmuReplay/Grid Code Check/Detect Event ==
  Vmeas : Inport
  Constant : Constant  Value=inLV_V(1)
  Constant1 : Constant  Value=inHV_V(1)
  Logical Operator : Logic  Operator=OR  AllPortsSameDT=off  OutDataTypeStr=boolean
  Relational Operator : RelationalOperator  Operator=<  OutDataTypeStr=boolean  RndMeth=Simplest
  Relational Operator1 : RelationalOperator  Operator=>  OutDataTypeStr=boolean  RndMeth=Simplest
  LV or HV Event : Outport
  wires:
  Vmeas/1 -> Relational Operator1/1, Relational Operator/1
  Constant/1 -> Relational Operator/2
  Logical Operator/1 -> LV or HV Event/1  "LV or HV Event"
  Constant1/1 -> Relational Operator1/2
  Relational Operator/1 -> Logical Operator/1  "LV Event"
  Relational Operator1/1 -> Logical Operator/2  "HV Event"

== system pmuReplay/Grid Code Check/Detect Event1 ==
  Vmeas : Inport
  Constant : Constant  Value=inLF_F(1)
  Constant1 : Constant  Value=inHF_F(1)
  Logical Operator : Logic  Operator=OR  AllPortsSameDT=off  OutDataTypeStr=boolean
  Relational Operator : RelationalOperator  Operator=<  OutDataTypeStr=boolean  RndMeth=Simplest
  Relational Operator1 : RelationalOperator  Operator=>  OutDataTypeStr=boolean  RndMeth=Simplest
  LF or HF Event : Outport
  wires:
  Relational Operator1/1 -> Logical Operator/2  "HF Event"
  Relational Operator/1 -> Logical Operator/1  "LF Event"
  Constant1/1 -> Relational Operator1/2
  Logical Operator/1 -> LF or HF Event/1
  Constant/1 -> Relational Operator/2
  Vmeas/1 -> Relational Operator/1, Relational Operator1/1

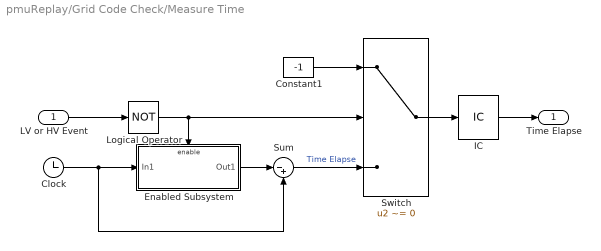
== system pmuReplay/Grid Code Check/Measure Time ==
  LV or HV Event : Inport
  Clock : Clock
  Constant1 : Constant  Value=-1
  Enabled Subsystem : Subsystem  TreatAsAtomicUnit=on
  IC : InitialCondition  Value=-1
  Logical Operator : Logic  Operator=NOT  AllPortsSameDT=off  OutDataTypeStr=boolean
  Sum : Sum  Inputs=|-+
  Switch : Switch  Criteria=u2 ~= 0
  Time Elapse : Outport
  wires:
  Enabled Subsystem/1(Out1) -> Sum/1
  Sum/1 -> Switch/3  "Time Elapse"
  Clock/1 -> Enabled Subsystem/1(In1), Sum/2
  Constant1/1 -> Switch/1
  Switch/1 -> IC/1
  LV or HV Event/1 -> Logical Operator/1
  Logical Operator/1 -> Switch/2, Enabled Subsystem/Enable
  IC/1 -> Time Elapse/1

== system pmuReplay/Grid Code Check/Minimum Event Time ==
  Time Elapse : Inport
  Compare To Constant : simulink/Logic and Bit Operations/Compare To Constant  relop=>  const=0  OutDataTypeStr=boolean
  Compare To Constant1 : simulink/Logic and Bit Operations/Compare To Constant  relop=<  const=resetTime  OutDataTypeStr=boolean
  Logical Operator1 : Logic  AllPortsSameDT=off  OutDataTypeStr=boolean
  CanReset : Outport
  wires:
  Time Elapse/1 -> Compare To Constant1/1, Compare To Constant/1
  Compare To Constant1/1 -> Logical Operator1/2
  Compare To Constant/1 -> Logical Operator1/1
  Logical Operator1/1 -> CanReset/1

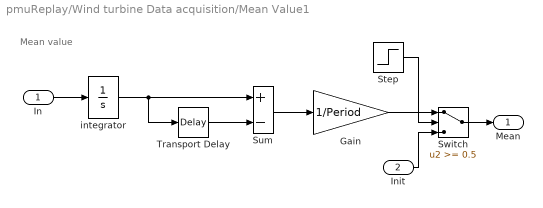
== system pmuReplay/Wind turbine Data acquisition/Mean Value1 ==
  note: Mean value
  In : Inport
  Init : Inport  Port=2
  Gain : Gain  Gain=1/Period  SaturateOnIntegerOverflow=on  OutDataTypeStr=Inherit: Same as input  ParamDataTypeStr=Inherit: Same as input
  Step : Step  Time=Period+eps  SampleTime=0
  Sum : Sum  Inputs=+-  SaturateOnIntegerOverflow=on  InputSameDT=on  OutDataTypeStr=Inherit: Same as first input
  Switch : Switch  Threshold=0.5  SaturateOnIntegerOverflow=on
  Transport Delay : TransportDelay  DelayTime=Period
  integrator : Integrator
  Mean : Outport
  wires:
  Transport Delay/1 -> Sum/2
  integrator/1 -> Transport Delay/1, Sum/1
  In/1 -> integrator/1
  Sum/1 -> Gain/1
  Gain/1 -> Switch/1
  Switch/1 -> Mean/1
  Step/1 -> Switch/2
  Init/1 -> Switch/3

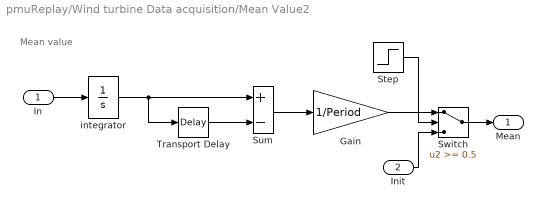
== system pmuReplay/Wind turbine Data acquisition/Mean Value2 ==
  note: Mean value
  In : Inport
  Init : Inport  Port=2
  Gain : Gain  Gain=1/Period  SaturateOnIntegerOverflow=on  OutDataTypeStr=Inherit: Same as input  ParamDataTypeStr=Inherit: Same as input
  Step : Step  Time=Period+eps  SampleTime=0
  Sum : Sum  Inputs=+-  SaturateOnIntegerOverflow=on  InputSameDT=on  OutDataTypeStr=Inherit: Same as first input
  Switch : Switch  Threshold=0.5  SaturateOnIntegerOverflow=on
  Transport Delay : TransportDelay  DelayTime=Period
  integrator : Integrator
  Mean : Outport
  wires:
  Init/1 -> Switch/3
  Step/1 -> Switch/2
  Switch/1 -> Mean/1
  Gain/1 -> Switch/1
  Sum/1 -> Gain/1
  In/1 -> integrator/1
  integrator/1 -> Sum/1, Transport Delay/1
  Transport Delay/1 -> Sum/2

== system pmuReplay/Wind turbine Data acquisition/Subsystem ==
  V (pu) : Inport
  Clock : Clock
  Compare To Constant : simulink/Logic and Bit Operations/Compare To Constant  relop=>=  const=5  OutDataTypeStr=boolean
  Constant2 : Constant
  Switch : Switch  Criteria=u2 > Threshold
  V : Outport
  wires:
  Clock/1 -> Compare To Constant/1
  Compare To Constant/1 -> Switch/2
  Switch/1 -> V/1
  Constant2/1 -> Switch/3
  V (pu)/1 -> Switch/1

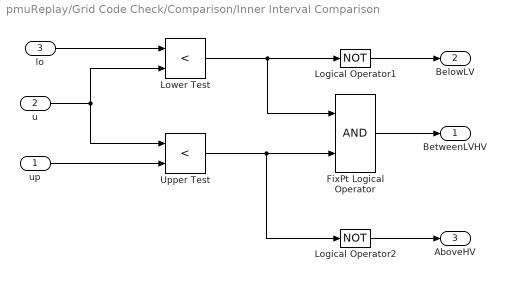
== system pmuReplay/Grid Code Check/Comparison/Inner Interval Comparison ==
  up : Inport
  u : Inport  Port=2
  lo : Inport  Port=3
  FixPt Logical Operator : Logic  AllPortsSameDT=off  OutDataTypeStr=boolean
  Logical Operator1 : Logic  Operator=NOT  AllPortsSameDT=off  OutDataTypeStr=boolean
  Logical Operator2 : Logic  Operator=NOT  AllPortsSameDT=off  OutDataTypeStr=boolean
  Lower Test : RelationalOperator  DisableCoverage=on  Operator=<  OutDataTypeStr=boolean  ZeroCross=off  RndMeth=Nearest
  Upper Test : RelationalOperator  DisableCoverage=on  Operator=<  OutDataTypeStr=boolean  ZeroCross=off  RndMeth=Nearest
  BetweenLVHV : Outport
  BelowLV : Outport  Port=2
  AboveHV : Outport  Port=3
  wires:
  Logical Operator2/1 -> AboveHV/1
  Logical Operator1/1 -> BelowLV/1
  lo/1 -> Lower Test/1
  up/1 -> Upper Test/2
  FixPt Logical Operator/1 -> BetweenLVHV/1
  Upper Test/1 -> FixPt Logical Operator/2, Logical Operator2/1
  Lower Test/1 -> FixPt Logical Operator/1, Logical Operator1/1
  u/1 -> Lower Test/2, Upper Test/1

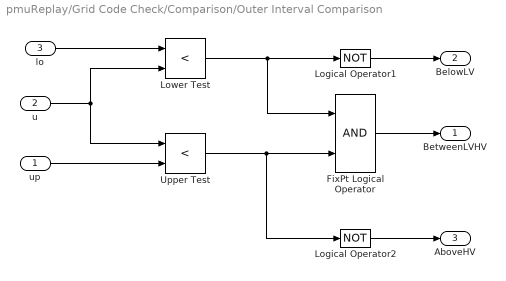
== system pmuReplay/Grid Code Check/Comparison/Outer Interval Comparison ==
  up : Inport
  u : Inport  Port=2
  lo : Inport  Port=3
  FixPt Logical Operator : Logic  AllPortsSameDT=off  OutDataTypeStr=boolean
  Logical Operator1 : Logic  Operator=NOT  AllPortsSameDT=off  OutDataTypeStr=boolean
  Logical Operator2 : Logic  Operator=NOT  AllPortsSameDT=off  OutDataTypeStr=boolean
  Lower Test : RelationalOperator  DisableCoverage=on  Operator=<  OutDataTypeStr=boolean  ZeroCross=off  RndMeth=Nearest
  Upper Test : RelationalOperator  DisableCoverage=on  Operator=<  OutDataTypeStr=boolean  ZeroCross=off  RndMeth=Nearest
  BetweenLVHV : Outport
  BelowLV : Outport  Port=2
  AboveHV : Outport  Port=3
  wires:
  u/1 -> Upper Test/1, Lower Test/2
  Lower Test/1 -> Logical Operator1/1, FixPt Logical Operator/1
  Upper Test/1 -> Logical Operator2/1, FixPt Logical Operator/2
  FixPt Logical Operator/1 -> BetweenLVHV/1
  up/1 -> Upper Test/2
  lo/1 -> Lower Test/1
  Logical Operator1/1 -> BelowLV/1
  Logical Operator2/1 -> AboveHV/1

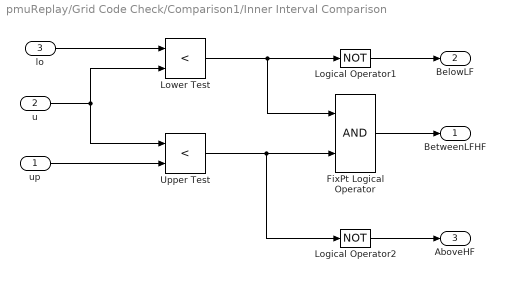
== system pmuReplay/Grid Code Check/Comparison1/Inner Interval Comparison ==
  up : Inport
  u : Inport  Port=2
  lo : Inport  Port=3
  FixPt Logical Operator : Logic  AllPortsSameDT=off  OutDataTypeStr=boolean
  Logical Operator1 : Logic  Operator=NOT  AllPortsSameDT=off  OutDataTypeStr=boolean
  Logical Operator2 : Logic  Operator=NOT  AllPortsSameDT=off  OutDataTypeStr=boolean
  Lower Test : RelationalOperator  DisableCoverage=on  Operator=<  OutDataTypeStr=boolean  ZeroCross=off  RndMeth=Nearest
  Upper Test : RelationalOperator  DisableCoverage=on  Operator=<  OutDataTypeStr=boolean  ZeroCross=off  RndMeth=Nearest
  BetweenLFHF : Outport
  BelowLF : Outport  Port=2
  AboveHF : Outport  Port=3
  wires:
  u/1 -> Upper Test/1, Lower Test/2
  Lower Test/1 -> Logical Operator1/1, FixPt Logical Operator/1
  Upper Test/1 -> Logical Operator2/1, FixPt Logical Operator/2
  FixPt Logical Operator/1 -> BetweenLFHF/1
  up/1 -> Upper Test/2
  lo/1 -> Lower Test/1
  Logical Operator1/1 -> BelowLF/1
  Logical Operator2/1 -> AboveHF/1

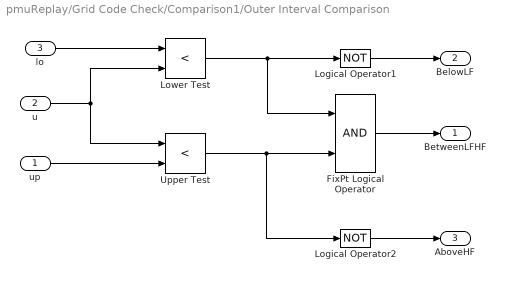
== system pmuReplay/Grid Code Check/Comparison1/Outer Interval Comparison ==
  up : Inport
  u : Inport  Port=2
  lo : Inport  Port=3
  FixPt Logical Operator : Logic  AllPortsSameDT=off  OutDataTypeStr=boolean
  Logical Operator1 : Logic  Operator=NOT  AllPortsSameDT=off  OutDataTypeStr=boolean
  Logical Operator2 : Logic  Operator=NOT  AllPortsSameDT=off  OutDataTypeStr=boolean
  Lower Test : RelationalOperator  DisableCoverage=on  Operator=<  OutDataTypeStr=boolean  ZeroCross=off  RndMeth=Nearest
  Upper Test : RelationalOperator  DisableCoverage=on  Operator=<  OutDataTypeStr=boolean  ZeroCross=off  RndMeth=Nearest
  BetweenLFHF : Outport
  BelowLF : Outport  Port=2
  AboveHF : Outport  Port=3
  wires:
  Logical Operator2/1 -> AboveHF/1
  Logical Operator1/1 -> BelowLF/1
  lo/1 -> Lower Test/1
  up/1 -> Upper Test/2
  FixPt Logical Operator/1 -> BetweenLFHF/1
  Upper Test/1 -> FixPt Logical Operator/2, Logical Operator2/1
  Lower Test/1 -> FixPt Logical Operator/1, Logical Operator1/1
  u/1 -> Lower Test/2, Upper Test/1

== system pmuReplay/Grid Code Check/Measure Time/Enabled Subsystem ==
  In1 : Inport
  Enable : EnablePort
  Out1 : Outport
  wires:
  In1/1 -> Out1/1

== matlab function pmuReplay/Plot 2D IEEE 1547-2018/MATLAB Function ==
  data: V input; F input; t input
function plotVF_1547(V,F,t)

persistent eventTime 
persistent mustPlot mayPlot vfPlot;

if isempty(eventTime)
    eventTime = 0;
end

% IEEE1547-2018 Values
IEEE1547.mayLVRT.T = [-1    0       0+1e-6  0.16  0.16+1e-6    10      10+1e-6     1000    1000+1e-6];
IEEE1547.mayLVRT.V = [0.88  0.88    0     0     0.45    0.45    0.7    0.7     0.88];
IEEE1547.mayHVRT.T = [-1    0	  0+1e-6     0.16     0.16+1e-6     10	10+1e-6	1000];
IEEE1547.mayHVRT.V = [1.1   1.1	  1.3   1.3      1.2      1.2	1.15	1.1];

IEEE1547.mustLVRT.T = [-1       0       0+1e-6     0.16     0.16+1e-6    0.32     0.32+1e-6    3       5        1000];
IEEE1547.mustLVRT.V = [0.88     0.88    0.3   0.3      0.45    0.45     0.65    0.65    0.88     0.88];
IEEE1547.mustHVRT.T = [-1	0	0+1e-6     0.2      0.2+1e-6     0.5	0.5+1e-6	1	1+1e-6	 600	600+1e-6];
IEEE1547.mustHVRT.V = [1.1	1.1	1.2   1.2      1.175   1.175	1.15	1.15	1.1	 1.1	1.1];

IEEE1547.mayLFRT.T = [-1, 0, 0+1e-6, 0.16-1e-6, 0.16, 300-1e-6, 300, 10000];
IEEE1547.mayLFRT.F = [58.5, 58.5, 50, 50, 56.5, 56.5, 58.5, 58.5];
IEEE1547.mayHFRT.T = [-1, 0, 0+1e-6, 0.16-1e-6, 0.16, 300-1e-6, 300, 1000-1e-6, 1000, 10000];
IEEE1547.mayHFRT.F = [60.6, 60.6, 66, 66, 62, 62, 61, 61, 60.6, 60.6];

IEEE1547.mustLFRT.T = [-1, 0, 0+1e-6, 299-1e-6, 299, 10000];
IEEE1547.mustLFRT.F = [58.5, 58.5, 57, 57, 58.5, 58.5];
IEEE1547.mustHFRT.T = [-1, 0, 0+1e-6, 299-1e-6, 299, 10000];
IEEE1547.mustHFRT.F = [60.6, 60.6, 62, 62, 60.6, 60.6];

if (V > 1.1 || V < 0.88 || F > 60.6 || F < 58.5) && eventTime == 0
    eventTime = t;
    diffTime = 1e-6;
elseif (t-eventTime) > 1000
    diffTime = 1e-6;
elseif eventTime > 0
    diffTime = t - eventTime;
else
    diffTime = 1e-6;
end

may.LV = interp1(IEEE1547.mayLVRT.T,IEEE1547.mayLVRT.V,diffTime);
may.HV = interp1(IEEE1547.mayHVRT.T,IEEE1547.mayHVRT.V,diffTime);
may.LF = interp1(IEEE1547.mayLFRT.T,IEEE1547.mayLFRT.F,diffTime);
may.HF = interp1(IEEE1547.mayHFRT.T,IEEE1547.mayHFRT.F,diffTime);
must.LV = interp1(IEEE1547.mustLVRT.T,IEEE1547.mustLVRT.V,diffTime);
must.HV = interp1(IEEE1547.mustHVRT.T,IEEE1547.mustHVRT.V,diffTime);
must.LF = interp1(IEEE1547.mustLFRT.T,IEEE1547.mustLFRT.F,diffTime);
must.HF = interp1(IEEE1547.mustHFRT.T,IEEE1547.mustHFRT.F,diffTime);

if isempty(mustPlot)
    figure(1); hold on;
    plot([58.5 60.6 60.6 58.5 58.5],[0.88 0.88 1.1 1.1 0.88],'Color',[0.2980    0.2980    0.2980],'LineWidth',2);
    mustPlot = plot([must.LF must.HF must.HF must.LF must.LF],...
        [must.LV must.LV must.HV must.HV must.LV],'Color',[0    0.5098    0.5569],'LineWidth',2);
    mayPlot = plot([may.LF may.HF may.HF may.LF may.LF],...
        [may.LV may.LV may.HV may.HV may.LV],'Color',[0.8941    0.5882    0],'LineWidth',2);
    plot([48 68 68 48 48],[0 0 1.5 1.5 0],'Color',[0.8824    0.5333    0.4627],'LineWidth',2);
    plot([60 60 NaN 48 68],[0 1.5 NaN 1 1],'LineStyle','-.','LineWidth',1,'Color','k');

    vfPlot = plot(F,V,'ro');
    
    hold off; grid on;
    xlim([48 68]);
    ylim([0 1.5]);
    
    xlabel('Frequency (Hz)'); ylabel('Voltage (pu)');
    title('IEEE 1547-2018 Ride Through Requirements');
else
    set(vfPlot,'XData',F,'YData',V);
    
    set(mustPlot,'XData',[must.LF must.HF must.HF must.LF must.LF],...
        'YData',[must.LV must.LV must.HV must.HV must.LV]);
    set(mayPlot,'XData',[may.LF may.HF may.HF may.LF may.LF],...
        'YData',[may.LV may.LV may.HV may.HV may.LV]);
    pause(0.01)
end
